simulink model "case3"  (R2024b)
settings: Solver=FixedStepAuto  StartTime=0  StopTime=1  FixedStep=1e-7  RelTol=1e-3
values from neighbouring files (symbols this model uses):
  SG_D_1_D = 0.01056    [IEEE9_case_parameters.m]    (also in case1_parameters.m; case2_parameters.m; case3_parameters.m; case4_parameters.m)
  SG_D_1_EnableSaturation = 0    [IEEE9_case_parameters.m]    (also in case1_parameters.m; case2_parameters.m; case3_parameters.m; case4_parameters.m)
  SG_D_1_f0 = 60    [IEEE9_case_parameters.m]    (also in case1_parameters.m; case2_parameters.m; case3_parameters.m; case4_parameters.m)
  SG_D_1_H = 7.5    [IEEE9_case_parameters.m]    (also in case1_parameters.m; case2_parameters.m; case3_parameters.m; case4_parameters.m)
  SG_D_1_K_A = 20    [IEEE9_case_parameters.m]    (also in case1_parameters.m; case2_parameters.m; case3_parameters.m; case4_parameters.m)
  SG_D_1_K_E = 1.000000e+1    (= 10)    [IEEE9_case_parameters.m]    (also in case1_parameters.m; case2_parameters.m; case3_parameters.m; case4_parameters.m)
  SG_D_1_K_F = 2.363    [IEEE9_case_parameters.m]    (also in case1_parameters.m; case2_parameters.m; case3_parameters.m; case4_parameters.m)
  SG_D_1_K_s = 0.5    [IEEE9_case_parameters.m]    (also in case1_parameters.m = 5; case2_parameters.m = 5; case3_parameters.m = 5; case4_parameters.m = 5)
  SG_D_1_R_a = 0.001088    [IEEE9_case_parameters.m]    (also in case1_parameters.m; case2_parameters.m; case3_parameters.m; case4_parameters.m)
  SG_D_1_S_A = 1    [IEEE9_case_parameters.m]    (also in case1_parameters.m; case2_parameters.m; case3_parameters.m; case4_parameters.m)
  SG_D_1_S_B = 0.103    [IEEE9_case_parameters.m]    (also in case1_parameters.m; case2_parameters.m; case3_parameters.m; case4_parameters.m)
  SG_D_1_S_N = 10.659857    [IEEE9_case_parameters.m]    (also in case1_parameters.m; case2_parameters.m; case3_parameters.m; case4_parameters.m)
  SG_D_1_SpeedPara = 200    [IEEE9_case_parameters.m]    (also in case1_parameters.m; case2_parameters.m; case3_parameters.m; case4_parameters.m)
  SG_D_1_T_0 = 0.720173    [IEEE9_case_parameters.m]    (also in case1_parameters.m = 0.755522; case2_parameters.m = 0.808931; case3_parameters.m = 0.869402; case4_parameters.m = 0.729316)
  SG_D_1_T_1 = 0.3    [IEEE9_case_parameters.m]    (also in case1_parameters.m; case2_parameters.m; case3_parameters.m; case4_parameters.m)
  SG_D_1_T_2 = 0.05    [IEEE9_case_parameters.m]    (also in case1_parameters.m; case2_parameters.m; case3_parameters.m; case4_parameters.m)
  SG_D_1_T_3 = 0.02    [IEEE9_case_parameters.m]    (also in case1_parameters.m; case2_parameters.m; case3_parameters.m; case4_parameters.m)
  SG_D_1_T_4 = 0.005    [IEEE9_case_parameters.m]    (also in case1_parameters.m; case2_parameters.m; case3_parameters.m; case4_parameters.m)
  SG_D_1_T_A = 0.02    [IEEE9_case_parameters.m]    (also in case1_parameters.m; case2_parameters.m; case3_parameters.m; case4_parameters.m)
  SG_D_1_T_dd = 8.000000e+0    (= 8)    [IEEE9_case_parameters.m]    (also in case1_parameters.m; case2_parameters.m; case3_parameters.m; case4_parameters.m)
  SG_D_1_T_ddd = 0.04    [IEEE9_case_parameters.m]    (also in case1_parameters.m; case2_parameters.m; case3_parameters.m; case4_parameters.m)
  SG_D_1_T_E = 0.314    [IEEE9_case_parameters.m]    (also in case1_parameters.m; case2_parameters.m; case3_parameters.m; case4_parameters.m)
  SG_D_1_T_F = 0.35    [IEEE9_case_parameters.m]    (also in case1_parameters.m; case2_parameters.m; case3_parameters.m; case4_parameters.m)
  SG_D_1_T_qd = 0.8    [IEEE9_case_parameters.m]    (also in case1_parameters.m; case2_parameters.m; case3_parameters.m; case4_parameters.m)
  SG_D_1_T_qdd = 0.02    [IEEE9_case_parameters.m]    (also in case1_parameters.m; case2_parameters.m; case3_parameters.m; case4_parameters.m)
  SG_D_1_T_speed = 0.1    [IEEE9_case_parameters.m]    (also in case1_parameters.m = 200; case2_parameters.m = 200; case3_parameters.m = 200; case4_parameters.m = 200)
  SG_D_1_T_w = 0.5    [IEEE9_case_parameters.m]    (also in case1_parameters.m; case2_parameters.m; case3_parameters.m; case4_parameters.m)
  SG_D_1_V_ref = 1.990276    [IEEE9_case_parameters.m]    (also in case1_parameters.m = 2.042296; case2_parameters.m = 2.051388; case3_parameters.m = 2.089584; case4_parameters.m = 2.01845)
  SG_D_1_w_ref = 376.991118    [IEEE9_case_parameters.m]    (also in case1_parameters.m; case2_parameters.m; case3_parameters.m; case4_parameters.m)
  SG_D_1_wb = 6.000000e+1    (= 60)    [IEEE9_case_parameters.m]    (also in case1_parameters.m; case2_parameters.m; case3_parameters.m; case4_parameters.m)
  SG_D_1_x_d = 1.9    [IEEE9_case_parameters.m]    (also in case1_parameters.m; case2_parameters.m; case3_parameters.m; case4_parameters.m)
  SG_D_1_x_dd = 0.302    [IEEE9_case_parameters.m]    (also in case1_parameters.m; case2_parameters.m; case3_parameters.m; case4_parameters.m)
  SG_D_1_x_ddd = 0.204    [IEEE9_case_parameters.m]    (also in case1_parameters.m; case2_parameters.m; case3_parameters.m; case4_parameters.m)
  SG_D_1_x_l = 0.05    [IEEE9_case_parameters.m]    (also in case1_parameters.m; case2_parameters.m; case3_parameters.m; case4_parameters.m)
  SG_D_1_x_q = 1.3    [IEEE9_case_parameters.m]    (also in case1_parameters.m; case2_parameters.m; case3_parameters.m; case4_parameters.m)
  SG_D_1_x_qd = 0.5    [IEEE9_case_parameters.m]    (also in case1_parameters.m; case2_parameters.m; case3_parameters.m; case4_parameters.m)
  SG_D_1_x_qdd = 0.3    [IEEE9_case_parameters.m]    (also in case1_parameters.m; case2_parameters.m; case3_parameters.m; case4_parameters.m)
  SG_D_2_D = 0.02    [IEEE9_case_parameters.m]    (also in case1_parameters.m; case2_parameters.m; case3_parameters.m; case4_parameters.m)
  SG_D_2_EnableSaturation = 0    [IEEE9_case_parameters.m]    (also in case1_parameters.m; case2_parameters.m; case3_parameters.m; case4_parameters.m)
  SG_D_2_f0 = 60    [IEEE9_case_parameters.m]    (also in case1_parameters.m; case2_parameters.m; case3_parameters.m; case4_parameters.m)
  SG_D_2_H = 8.000000e+0    (= 8)    [IEEE9_case_parameters.m]    (also in case1_parameters.m; case2_parameters.m; case3_parameters.m; case4_parameters.m)
  SG_D_2_K_A = 20    [IEEE9_case_parameters.m]    (also in case1_parameters.m; case2_parameters.m; case3_parameters.m; case4_parameters.m)
  SG_D_2_K_E = 1.000000e+1    (= 10)    [IEEE9_case_parameters.m]    (also in case1_parameters.m; case2_parameters.m; case3_parameters.m; case4_parameters.m)
  SG_D_2_K_F = 2.363    [IEEE9_case_parameters.m]    (also in case1_parameters.m; case2_parameters.m; case3_parameters.m; case4_parameters.m)
  SG_D_2_K_s = 0.5    [IEEE9_case_parameters.m]    (also in case1_parameters.m = 4; case2_parameters.m = 4; case3_parameters.m = 4; case4_parameters.m = 4)
  SG_D_2_R_a = 0.001088    [IEEE9_case_parameters.m]    (also in case1_parameters.m; case2_parameters.m; case3_parameters.m; case4_parameters.m)
  SG_D_2_S_A = 1    [IEEE9_case_parameters.m]    (also in case1_parameters.m; case2_parameters.m; case3_parameters.m; case4_parameters.m)
  SG_D_2_S_B = 0.103    [IEEE9_case_parameters.m]    (also in case1_parameters.m; case2_parameters.m; case3_parameters.m; case4_parameters.m)
  SG_D_2_S_N = 10.659857    [IEEE9_case_parameters.m]    (also in case1_parameters.m; case2_parameters.m; case3_parameters.m; case4_parameters.m)
  SG_D_2_SpeedPara = 200    [IEEE9_case_parameters.m]    (also in case1_parameters.m; case2_parameters.m; case3_parameters.m; case4_parameters.m)
  SG_D_2_T_0 = 1.632913    [IEEE9_case_parameters.m]    (also in case1_parameters.m = 1.632925; case2_parameters.m = 1.632915; case3_parameters.m = 1.632914; case4_parameters.m = 1.632927)
  SG_D_2_T_1 = 0.2    [IEEE9_case_parameters.m]    (also in case1_parameters.m; case2_parameters.m; case3_parameters.m; case4_parameters.m)
  SG_D_2_T_2 = 0.05    [IEEE9_case_parameters.m]    (also in case1_parameters.m; case2_parameters.m; case3_parameters.m; case4_parameters.m)
  SG_D_2_T_3 = 0.02    [IEEE9_case_parameters.m]    (also in case1_parameters.m; case2_parameters.m; case3_parameters.m; case4_parameters.m)
  SG_D_2_T_4 = 0.005    [IEEE9_case_parameters.m]    (also in case1_parameters.m; case2_parameters.m; case3_parameters.m; case4_parameters.m)
  SG_D_2_T_A = 0.02    [IEEE9_case_parameters.m]    (also in case1_parameters.m; case2_parameters.m; case3_parameters.m; case4_parameters.m)
  SG_D_2_T_dd = 7.9    [IEEE9_case_parameters.m]    (also in case1_parameters.m; case2_parameters.m; case3_parameters.m; case4_parameters.m)
  SG_D_2_T_ddd = 0.04    [IEEE9_case_parameters.m]    (also in case1_parameters.m; case2_parameters.m; case3_parameters.m; case4_parameters.m)
  SG_D_2_T_E = 0.314    [IEEE9_case_parameters.m]    (also in case1_parameters.m; case2_parameters.m; case3_parameters.m; case4_parameters.m)
  SG_D_2_T_F = 0.35    [IEEE9_case_parameters.m]    (also in case1_parameters.m; case2_parameters.m; case3_parameters.m; case4_parameters.m)
  SG_D_2_T_qd = 0.8    [IEEE9_case_parameters.m]    (also in case1_parameters.m; case2_parameters.m; case3_parameters.m; case4_parameters.m)
  SG_D_2_T_qdd = 0.015    [IEEE9_case_parameters.m]    (also in case1_parameters.m; case2_parameters.m; case3_parameters.m; case4_parameters.m)
  SG_D_2_T_speed = 0.1    [IEEE9_case_parameters.m]    (also in case1_parameters.m = 150; case2_parameters.m = 150; case3_parameters.m = 150; case4_parameters.m = 150)
  SG_D_2_T_w = 0.35    [IEEE9_case_parameters.m]    (also in case1_parameters.m; case2_parameters.m; case3_parameters.m; case4_parameters.m)
  SG_D_2_V_ref = 2.58547    [IEEE9_case_parameters.m]    (also in case1_parameters.m = 2.597896; case2_parameters.m = 2.587136; case3_parameters.m = 2.586042; case4_parameters.m = 2.599679)
  SG_D_2_w_ref = 376.991118    [IEEE9_case_parameters.m]    (also in case1_parameters.m; case2_parameters.m; case3_parameters.m; case4_parameters.m)
  SG_D_2_wb = 6.000000e+1    (= 60)    [IEEE9_case_parameters.m]    (also in case1_parameters.m; case2_parameters.m; case3_parameters.m; case4_parameters.m)
  SG_D_2_x_d = 1.8    [IEEE9_case_parameters.m]    (also in case1_parameters.m; case2_parameters.m; case3_parameters.m; case4_parameters.m)
  SG_D_2_x_dd = 0.302    [IEEE9_case_parameters.m]    (also in case1_parameters.m; case2_parameters.m; case3_parameters.m; case4_parameters.m)
  SG_D_2_x_ddd = 0.204    [IEEE9_case_parameters.m]    (also in case1_parameters.m; case2_parameters.m; case3_parameters.m; case4_parameters.m)
  SG_D_2_x_l = 0.05    [IEEE9_case_parameters.m]    (also in case1_parameters.m; case2_parameters.m; case3_parameters.m; case4_parameters.m)
  SG_D_2_x_q = 1.25    [IEEE9_case_parameters.m]    (also in case1_parameters.m; case2_parameters.m; case3_parameters.m; case4_parameters.m)
  SG_D_2_x_qd = 0.5    [IEEE9_case_parameters.m]    (also in case1_parameters.m; case2_parameters.m; case3_parameters.m; case4_parameters.m)
  SG_D_2_x_qdd = 0.3    [IEEE9_case_parameters.m]    (also in case1_parameters.m; case2_parameters.m; case3_parameters.m; case4_parameters.m)
  SG_D_3_D = 0.02    [IEEE9_case_parameters.m]    (also in case1_parameters.m; case2_parameters.m; case3_parameters.m; case4_parameters.m)
  SG_D_3_EnableSaturation = 0    [IEEE9_case_parameters.m]    (also in case1_parameters.m; case2_parameters.m; case3_parameters.m; case4_parameters.m)
  SG_D_3_f0 = 60    [IEEE9_case_parameters.m]    (also in case1_parameters.m; case2_parameters.m; case3_parameters.m; case4_parameters.m)
  SG_D_3_H = 7.7    [IEEE9_case_parameters.m]    (also in case1_parameters.m; case2_parameters.m; case3_parameters.m; case4_parameters.m)
  SG_D_3_K_A = 20    [IEEE9_case_parameters.m]    (also in case1_parameters.m; case2_parameters.m; case3_parameters.m; case4_parameters.m)
  SG_D_3_K_E = 1.000000e+1    (= 10)    [IEEE9_case_parameters.m]    (also in case1_parameters.m; case2_parameters.m; case3_parameters.m; case4_parameters.m)
  SG_D_3_K_F = 2.363    [IEEE9_case_parameters.m]    (also in case1_parameters.m; case2_parameters.m; case3_parameters.m; case4_parameters.m)
  SG_D_3_K_s = 0.2    [IEEE9_case_parameters.m]    (also in case1_parameters.m = 2; case2_parameters.m = 2; case3_parameters.m = 2; case4_parameters.m = 2)
  SG_D_3_R_a = 0.001088    [IEEE9_case_parameters.m]    (also in case1_parameters.m; case2_parameters.m; case3_parameters.m; case4_parameters.m)
  SG_D_3_S_A = 1    [IEEE9_case_parameters.m]    (also in case1_parameters.m; case2_parameters.m; case3_parameters.m; case4_parameters.m)
  SG_D_3_S_B = 0.103    [IEEE9_case_parameters.m]    (also in case1_parameters.m; case2_parameters.m; case3_parameters.m; case4_parameters.m)
  SG_D_3_S_N = 10.659857    [IEEE9_case_parameters.m]    (also in case1_parameters.m; case2_parameters.m; case3_parameters.m; case4_parameters.m)
  SG_D_3_SpeedPara = 200    [IEEE9_case_parameters.m]    (also in case1_parameters.m; case2_parameters.m; case3_parameters.m; case4_parameters.m)
  SG_D_3_T_0 = 0.850788    [IEEE9_case_parameters.m]    (also in case1_parameters.m = 0.850786; case2_parameters.m = 0.850787; case3_parameters.m; case4_parameters.m = 0.850786)
  SG_D_3_T_1 = 0.2    [IEEE9_case_parameters.m]    (also in case1_parameters.m; case2_parameters.m; case3_parameters.m; case4_parameters.m)
  SG_D_3_T_2 = 0.05    [IEEE9_case_parameters.m]    (also in case1_parameters.m; case2_parameters.m; case3_parameters.m; case4_parameters.m)
  SG_D_3_T_3 = 0.02    [IEEE9_case_parameters.m]    (also in case1_parameters.m; case2_parameters.m; case3_parameters.m; case4_parameters.m)
  SG_D_3_T_4 = 0.005    [IEEE9_case_parameters.m]    (also in case1_parameters.m; case2_parameters.m; case3_parameters.m; case4_parameters.m)
  SG_D_3_T_A = 0.02    [IEEE9_case_parameters.m]    (also in case1_parameters.m; case2_parameters.m; case3_parameters.m; case4_parameters.m)
  SG_D_3_T_dd = 8.1    [IEEE9_case_parameters.m]    (also in case1_parameters.m; case2_parameters.m; case3_parameters.m; case4_parameters.m)
  SG_D_3_T_ddd = 0.04    [IEEE9_case_parameters.m]    (also in case1_parameters.m; case2_parameters.m; case3_parameters.m; case4_parameters.m)
  SG_D_3_T_E = 0.314    [IEEE9_case_parameters.m]    (also in case1_parameters.m; case2_parameters.m; case3_parameters.m; case4_parameters.m)
  SG_D_3_T_F = 0.35    [IEEE9_case_parameters.m]    (also in case1_parameters.m; case2_parameters.m; case3_parameters.m; case4_parameters.m)
  SG_D_3_T_qd = 0.8    [IEEE9_case_parameters.m]    (also in case1_parameters.m; case2_parameters.m; case3_parameters.m; case4_parameters.m)
  SG_D_3_T_qdd = 0.015    [IEEE9_case_parameters.m]    (also in case1_parameters.m; case2_parameters.m; case3_parameters.m; case4_parameters.m)
  SG_D_3_T_speed = 0.1    [IEEE9_case_parameters.m]    (also in case1_parameters.m = 180; case2_parameters.m = 180; case3_parameters.m = 180; case4_parameters.m = 180)
  SG_D_3_T_w = 0.4    [IEEE9_case_parameters.m]    (also in case1_parameters.m; case2_parameters.m; case3_parameters.m; case4_parameters.m)
  SG_D_3_V_ref = 1.892727    [IEEE9_case_parameters.m]    (also in case1_parameters.m = 1.906439; case2_parameters.m = 1.895535; case3_parameters.m = 1.892105; case4_parameters.m = 1.906598)
  SG_D_3_w_ref = 376.991118    [IEEE9_case_parameters.m]    (also in case1_parameters.m; case2_parameters.m; case3_parameters.m; case4_parameters.m)
  SG_D_3_wb = 6.000000e+1    (= 60)    [IEEE9_case_parameters.m]    (also in case1_parameters.m; case2_parameters.m; case3_parameters.m; case4_parameters.m)
  SG_D_3_x_d = 1.85    [IEEE9_case_parameters.m]    (also in case1_parameters.m; case2_parameters.m; case3_parameters.m; case4_parameters.m)
  SG_D_3_x_dd = 0.302    [IEEE9_case_parameters.m]    (also in case1_parameters.m; case2_parameters.m; case3_parameters.m; case4_parameters.m)
  SG_D_3_x_ddd = 0.204    [IEEE9_case_parameters.m]    (also in case1_parameters.m; case2_parameters.m; case3_parameters.m; case4_parameters.m)
  SG_D_3_x_l = 0.05    [IEEE9_case_parameters.m]    (also in case1_parameters.m; case2_parameters.m; case3_parameters.m; case4_parameters.m)
  SG_D_3_x_q = 1.2    [IEEE9_case_parameters.m]    (also in case1_parameters.m; case2_parameters.m; case3_parameters.m; case4_parameters.m)
  SG_D_3_x_qd = 0.5    [IEEE9_case_parameters.m]    (also in case1_parameters.m; case2_parameters.m; case3_parameters.m; case4_parameters.m)
  SG_D_3_x_qdd = 0.3    [IEEE9_case_parameters.m]    (also in case1_parameters.m; case2_parameters.m; case3_parameters.m; case4_parameters.m)
(part 7 of 12)

== system case3/SG_D_2/T_e_SG_D_2_block ==
  note: T_e_SG_D_2 in case3
      | $-\frac{\psi _{d,\mathrm{SG},D,2}\,\left(\psi _{q,\mathrm{SG},D,2}+\frac{\psi _{\mathrm{gq},\mathrm{SG},D,2}\,\left(x_{l}-x_{\mathrm{qdd}}\right)}{x_{l}-x_{\mathrm{qd}}}+\frac{\psi _{\mathrm{kq},\mathrm{SG},D,2}\,\left(x_{\mathrm{qd}}-x_{\mathrm{qdd}}\right)}{x_{l}-x_{\mathrm{qd}}}\right)}{x_{\mathrm{qdd}}}-\frac{\psi _{q,\mathrm{SG},D,2}\,\left(\frac{\psi _{\mathrm{1d},\mathrm{SG},D,2}\,\left(x_{\mathrm{dd}}-x_{\mathrm{ddd}}\right)}{x_{\mathrm{dd}}-x_{l}}-\psi _{d,\mathrm{SG},D,2}+\frac{\psi _{\mathrm{fd},\mathrm{SG},D,2}\,\left(x_{\mathrm{ddd}}-x_{l}\right)}{x_{\mathrm{dd}}-x_{l}}\right)}{x_{\mathrm{ddd}}}$
      | Automatically generated on 2025-10-31 19:00:41 .
  State_psi_d_SG_D_2_bd8f2 : Inport
  State_psi_gq_SG_D_2_7cf1b : Inport  Port=2
  State_psi_kq_SG_D_2_00a62 : Inport  Port=3
  State_psi_q_SG_D_2_fc5b5 : Inport  Port=4
  State_psi_q_SG_D_2_0409e : Inport  Port=5
  State_psi_1d_SG_D_2_3067b : Inport  Port=6
  State_psi_d_SG_D_2_0f14f : Inport  Port=7
  State_psi_fd_SG_D_2_e1184 : Inport  Port=8
  Add_1d177 : Sum
  Add_42747 : Sum
  Add_5d270 : Sum
  Add_b1493 : Sum
  Add_c9106 : Sum
  Add_e7ab1 : Sum
  Constant_-1_0d88f : Constant  Value=-1
  Constant_-1_2e7fe : Constant  Value=-1
  Constant_-1_4cbe8 : Constant  Value=-1
  Constant_-1_6ebdc : Constant  Value=-1
  Constant_-1_f2e90 : Constant  Value=-1
  Constant_x_dd_7ba48 : Constant  Value=x_dd
  Constant_x_dd_9e0e7 : Constant  Value=x_dd
  Constant_x_dd_a49ec : Constant  Value=x_dd
  Constant_x_ddd_3889b : Constant  Value=x_ddd
  Constant_x_ddd_8a46c : Constant  Value=x_ddd
  Constant_x_ddd_f7651 : Constant  Value=x_ddd
  Constant_x_l_2e2bb : Constant  Value=x_l
  Constant_x_l_3f6eb : Constant  Value=x_l
  Constant_x_l_47e81 : Constant  Value=x_l
  Constant_x_l_4ea90 : Constant  Value=x_l
  Constant_x_l_7f158 : Constant  Value=x_l
  Constant_x_l_d88ad : Constant  Value=x_l
  Constant_x_qd_2c9ed : Constant  Value=x_qd
  Constant_x_qd_5af5b : Constant  Value=x_qd
  Constant_x_qd_fa8b9 : Constant  Value=x_qd
  Constant_x_qdd_6bb06 : Constant  Value=x_qdd
  Constant_x_qdd_71248 : Constant  Value=x_qdd
  Constant_x_qdd_ce159 : Constant  Value=x_qdd
  Divide_3e111 : Product  Inputs=*/
  Divide_4e959 : Product  Inputs=*/
  Divide_66ff5 : Product  Inputs=*/
  Divide_7bee8 : Product  Inputs=*/
  Divide_7d3ab : Product  Inputs=*/
  Divide_8540e : Product  Inputs=*/
  Product_2024f : Product
  Product_2debf : Product
  Product_312dd : Product
  Product_42b1c : Product
  Product_56005 : Product
  Product_711bf : Product
  Product_73a18 : Product
  Product_b399e : Product
  Product_bcb12 : Product
  Product_e72c3 : Product
  Product_f0df5 : Product
  Subtract_1307a : Sum  Inputs=+-
  Subtract_1559b : Sum  Inputs=+-
  Subtract_45dc1 : Sum  Inputs=+-
  Subtract_73649 : Sum  Inputs=+-
  Subtract_9e724 : Sum  Inputs=+-
  Subtract_cfab8 : Sum  Inputs=+-
  Subtract_da0d6 : Sum  Inputs=+-
  Blockout_T_e_SG_D_2_f9887 : Outport
  wires:
  Constant_-1_6ebdc/1 -> Product_bcb12/1
  Divide_7d3ab/1 -> Subtract_cfab8/1
  Constant_-1_4cbe8/1 -> Product_73a18/1
  Constant_x_l_3f6eb/1 -> Product_73a18/2
  Constant_x_qd_5af5b/1 -> Subtract_da0d6/1
  Product_e72c3/1 -> Divide_7d3ab/1
  Product_73a18/1 -> Add_e7ab1/1
  Divide_7bee8/1 -> Subtract_9e724/2
  Constant_x_qdd_71248/1 -> Subtract_da0d6/2
  Constant_x_qdd_6bb06/1 -> Divide_66ff5/2
  Constant_x_ddd_8a46c/1 -> Subtract_73649/2
  Constant_x_qdd_ce159/1 -> Add_e7ab1/2
  Constant_x_l_47e81/1 -> Product_bcb12/2
  Constant_-1_f2e90/1 -> Product_2debf/1
  Constant_x_l_7f158/1 -> Product_2debf/2
  Constant_-1_0d88f/1 -> Product_b399e/1
  State_psi_1d_SG_D_2_3067b/1 -> Product_b399e/2
  Constant_x_dd_9e0e7/1 -> Subtract_73649/1
  Divide_8540e/1 -> Subtract_cfab8/2
  State_psi_gq_SG_D_2_7cf1b/1 -> Product_e72c3/1
  Add_e7ab1/1 -> Product_e72c3/2
  Subtract_cfab8/1 -> Add_5d270/1
  Constant_x_dd_7ba48/1 -> Subtract_45dc1/1
  Product_bcb12/1 -> Add_c9106/1
  Product_56005/1 -> Product_2024f/1
  Constant_x_qd_fa8b9/1 -> Add_c9106/2
  State_psi_kq_SG_D_2_00a62/1 -> Product_312dd/1
  Subtract_da0d6/1 -> Product_312dd/2
  Product_2debf/1 -> Add_b1493/1
  State_psi_q_SG_D_2_0409e/1 -> Product_42b1c/1
  Constant_x_qd_2c9ed/1 -> Add_b1493/2
  Product_b399e/1 -> Product_711bf/1
  Divide_4e959/1 -> Add_42747/2
  Subtract_73649/1 -> Product_711bf/2
  Constant_x_l_d88ad/1 -> Subtract_45dc1/2
  Constant_x_ddd_3889b/1 -> Subtract_1307a/1
  Constant_x_dd_a49ec/1 -> Subtract_1559b/1
  Constant_x_l_2e2bb/1 -> Subtract_1307a/2
  Add_42747/1 -> Blockout_T_e_SG_D_2_f9887/1
  Add_c9106/1 -> Divide_7d3ab/2
  Product_312dd/1 -> Divide_8540e/1
  Product_2024f/1 -> Divide_66ff5/1
  State_psi_d_SG_D_2_bd8f2/1 -> Product_56005/2
  Add_b1493/1 -> Divide_8540e/2
  Product_711bf/1 -> Divide_3e111/1
  Subtract_45dc1/1 -> Divide_3e111/2
  Constant_x_l_4ea90/1 -> Subtract_1559b/2
  State_psi_fd_SG_D_2_e1184/1 -> Product_f0df5/1
  Constant_x_ddd_f7651/1 -> Divide_4e959/2
  Product_42b1c/1 -> Divide_4e959/1
  Subtract_1307a/1 -> Product_f0df5/2
  Divide_3e111/1 -> Add_1d177/1
  State_psi_d_SG_D_2_0f14f/1 -> Add_1d177/2
  Add_1d177/1 -> Subtract_9e724/1
  Product_f0df5/1 -> Divide_7bee8/1
  Subtract_1559b/1 -> Divide_7bee8/2
  Constant_-1_2e7fe/1 -> Product_56005/1
  State_psi_q_SG_D_2_fc5b5/1 -> Add_5d270/2
  Add_5d270/1 -> Product_2024f/2
  Subtract_9e724/1 -> Product_42b1c/2
  Divide_66ff5/1 -> Add_42747/1

== system case3/SG_D_2/d_E_fd_SG_D_2_block ==
  note: d_E_fd_SG_D_2 in case3
      | $\frac{V_{f,\mathrm{SG},D,2}-E_{\mathrm{fd},\mathrm{SG},D,2}\,K_{E}}{T_{E}}$
      | Automatically generated on 2025-10-31 19:00:25 .
  State_E_fd_SG_D_2_aeb78 : Inport
  State_V_f_SG_D_2_75a88 : Inport  Port=2
  Add_3aad2 : Sum
  Constant_-1_2bcf9 : Constant  Value=-1
  Constant_K_E_34ed1 : Constant  Value=K_E
  Constant_T_E_1a99d : Constant  Value=T_E
  Divide_16824 : Product  Inputs=*/
  Product_22060 : Product
  Product_ea532 : Product
  Blockout_d_E_fd_SG_D_2_c4f8a : Outport
  wires:
  Constant_-1_2bcf9/1 -> Product_ea532/1
  State_E_fd_SG_D_2_aeb78/1 -> Product_ea532/2
  Product_ea532/1 -> Product_22060/1
  Constant_K_E_34ed1/1 -> Product_22060/2
  Product_22060/1 -> Add_3aad2/1
  Constant_T_E_1a99d/1 -> Divide_16824/2
  State_V_f_SG_D_2_75a88/1 -> Add_3aad2/2
  Add_3aad2/1 -> Divide_16824/1
  Divide_16824/1 -> Blockout_d_E_fd_SG_D_2_c4f8a/1

== system case3/SG_D_2/d_Px_1_SG_D_2_block ==
  note: d_Px_1_SG_D_2 in case3
      | $\frac{w_{\mathrm{SG},D,2}-2\,\pi \,f_{0}}{T_{w}}-\frac{\mathrm{Px}_{1,\mathrm{SG},D,2}}{T_{w}}$
      | Automatically generated on 2025-10-31 19:00:26 .
  State_Px_1_SG_D_2_e1673 : Inport
  State_w_SG_D_2_bbb39 : Inport  Port=2
  Add_08d45 : Sum
  Add_4d18d : Sum
  Constant_-1_0bff0 : Constant  Value=-1
  Constant_-2.0_0421e : Constant  Value=-2.0
  Constant_T_w_34646 : Constant  Value=T_w
  Constant_T_w_c89ad : Constant  Value=T_w
  Constant_f0_04b6a : Constant  Value=f0
  Constant_pi_beef7 : Constant  Value=pi
  Divide_48226 : Product  Inputs=*/
  Divide_d9862 : Product  Inputs=*/
  Product_7dcbd : Product
  Product_cef66 : Product
  Product_ec7ca : Product
  Blockout_d_Px_1_SG_D_2_109b7 : Outport
  wires:
  Constant_-2.0_0421e/1 -> Product_7dcbd/1
  State_w_SG_D_2_bbb39/1 -> Add_4d18d/2
  Constant_pi_beef7/1 -> Product_7dcbd/2
  Product_7dcbd/1 -> Product_ec7ca/1
  Constant_f0_04b6a/1 -> Product_ec7ca/2
  Constant_-1_0bff0/1 -> Product_cef66/1
  State_Px_1_SG_D_2_e1673/1 -> Product_cef66/2
  Product_ec7ca/1 -> Add_4d18d/1
  Product_cef66/1 -> Divide_48226/1
  Constant_T_w_c89ad/1 -> Divide_48226/2
  Add_4d18d/1 -> Divide_d9862/1
  Constant_T_w_34646/1 -> Divide_d9862/2
  Divide_48226/1 -> Add_08d45/1
  Divide_d9862/1 -> Add_08d45/2
  Add_08d45/1 -> Blockout_d_Px_1_SG_D_2_109b7/1

== system case3/SG_D_2/d_Px_2_SG_D_2_block ==
  note: d_Px_2_SG_D_2 in case3
      | $\frac{\mathrm{Px}_{1,\mathrm{SG},D,2}-T_{2}\,\left(\frac{\mathrm{Px}_{1,\mathrm{SG},D,2}}{T_{w}}-\frac{w_{\mathrm{SG},D,2}-2\,\pi \,f_{0}}{T_{w}}\right)}{T_{1}}-\frac{\mathrm{Px}_{2,\mathrm{SG},D,2}}{T_{1}}$
      | Automatically generated on 2025-10-31 19:00:27 .
  State_Px_2_SG_D_2_a9fab : Inport
  State_Px_1_SG_D_2_b7eac : Inport  Port=2
  State_Px_1_SG_D_2_ca2a4 : Inport  Port=3
  State_w_SG_D_2_0d46f : Inport  Port=4
  Add_05522 : Sum
  Add_5cdaa : Sum
  Add_6c463 : Sum
  Add_d61f3 : Sum
  Constant_-1_14cce : Constant  Value=-1
  Constant_-1_44d6b : Constant  Value=-1
  Constant_-2.0_02914 : Constant  Value=-2.0
  Constant_T_1_53e96 : Constant  Value=T_1
  Constant_T_1_a5862 : Constant  Value=T_1
  Constant_T_2_b2b5a : Constant  Value=T_2
  Constant_T_w_a3a65 : Constant  Value=T_w
  Constant_T_w_e47eb : Constant  Value=T_w
  Constant_f0_8ff7e : Constant  Value=f0
  Constant_pi_131b0 : Constant  Value=pi
  Divide_9619a : Product  Inputs=*/
  Divide_a2959 : Product  Inputs=*/
  Divide_bb976 : Product  Inputs=*/
  Divide_df334 : Product  Inputs=*/
  Product_334ce : Product
  Product_6f84f : Product
  Product_de7e1 : Product
  Product_ed4b0 : Product
  Product_f3691 : Product
  Blockout_d_Px_2_SG_D_2_1ade1 : Outport
  wires:
  Constant_-1_14cce/1 -> Product_334ce/1
  Constant_-2.0_02914/1 -> Product_de7e1/1
  Product_f3691/1 -> Add_5cdaa/2
  State_w_SG_D_2_0d46f/1 -> Add_6c463/2
  Constant_pi_131b0/1 -> Product_de7e1/2
  Product_de7e1/1 -> Product_ed4b0/1
  State_Px_1_SG_D_2_ca2a4/1 -> Product_6f84f/2
  Constant_f0_8ff7e/1 -> Product_ed4b0/2
  State_Px_2_SG_D_2_a9fab/1 -> Product_334ce/2
  Constant_-1_44d6b/1 -> Product_6f84f/1
  Product_ed4b0/1 -> Add_6c463/1
  Product_6f84f/1 -> Divide_a2959/1
  Constant_T_w_a3a65/1 -> Divide_a2959/2
  Add_6c463/1 -> Divide_9619a/1
  Constant_T_w_e47eb/1 -> Divide_9619a/2
  Divide_a2959/1 -> Add_05522/1
  Divide_9619a/1 -> Add_05522/2
  Constant_T_2_b2b5a/1 -> Product_f3691/1
  Add_05522/1 -> Product_f3691/2
  State_Px_1_SG_D_2_b7eac/1 -> Add_5cdaa/1
  Product_334ce/1 -> Divide_df334/1
  Constant_T_1_a5862/1 -> Divide_df334/2
  Add_5cdaa/1 -> Divide_bb976/1
  Constant_T_1_53e96/1 -> Divide_bb976/2
  Divide_df334/1 -> Add_d61f3/1
  Divide_bb976/1 -> Add_d61f3/2
  Add_d61f3/1 -> Blockout_d_Px_2_SG_D_2_1ade1/1

== system case3/SG_D_2/d_Px_3_SG_D_2_block ==
  note: d_Px_3_SG_D_2 in case3
      | $\frac{\mathrm{Px}_{2,\mathrm{SG},D,2}+T_{4}\,\left(\frac{\mathrm{Px}_{1,\mathrm{SG},D,2}-T_{2}\,\left(\frac{\mathrm{Px}_{1,\mathrm{SG},D,2}}{T_{w}}-\frac{w_{\mathrm{SG},D,2}-2\,\pi \,f_{0}}{T_{w}}\right)}{T_{1}}-\frac{\mathrm{Px}_{2,\mathrm{SG},D,2}}{T_{1}}\right)}{T_{3}}-\frac{\mathrm{Px}_{3,\mathrm{SG},D,2}}{T_{3}}$
      | Automatically generated on 2025-10-31 19:00:30 .
  State_Px_3_SG_D_2_127e3 : Inport
  State_Px_2_SG_D_2_c1187 : Inport  Port=2
  State_Px_2_SG_D_2_e6f9b : Inport  Port=3
  State_Px_1_SG_D_2_d9778 : Inport  Port=4
  State_Px_1_SG_D_2_e27f8 : Inport  Port=5
  State_w_SG_D_2_22dc6 : Inport  Port=6
  Add_0cd75 : Sum
  Add_9f753 : Sum
  Add_ad80e : Sum
  Add_bc041 : Sum
  Add_d454c : Sum
  Add_e63a9 : Sum
  Constant_-1_07edb : Constant  Value=-1
  Constant_-1_13db9 : Constant  Value=-1
  Constant_-1_77d78 : Constant  Value=-1
  Constant_-2.0_d8f8b : Constant  Value=-2.0
  Constant_T_1_8ecf8 : Constant  Value=T_1
  Constant_T_1_fad53 : Constant  Value=T_1
  Constant_T_2_f64fd : Constant  Value=T_2
  Constant_T_3_52c41 : Constant  Value=T_3
  Constant_T_3_a0ec5 : Constant  Value=T_3
  Constant_T_4_606e5 : Constant  Value=T_4
  Constant_T_w_319fe : Constant  Value=T_w
  Constant_T_w_36f52 : Constant  Value=T_w
  Constant_f0_07c30 : Constant  Value=f0
  Constant_pi_a9680 : Constant  Value=pi
  Divide_5bcdb : Product  Inputs=*/
  Divide_6b17f : Product  Inputs=*/
  Divide_ba923 : Product  Inputs=*/
  Divide_beeaf : Product  Inputs=*/
  Divide_c57bf : Product  Inputs=*/
  Divide_f497b : Product  Inputs=*/
  Product_147fa : Product
  Product_201e1 : Product
  Product_24bd8 : Product
  Product_26550 : Product
  Product_2e2b4 : Product
  Product_4511e : Product
  Product_f1616 : Product
  Blockout_d_Px_3_SG_D_2_2b25a : Outport
  wires:
  Constant_-2.0_d8f8b/1 -> Product_4511e/1
  State_w_SG_D_2_22dc6/1 -> Add_ad80e/2
  Add_d454c/1 -> Divide_6b17f/1
  Constant_pi_a9680/1 -> Product_4511e/2
  Constant_-1_07edb/1 -> Product_201e1/1
  Product_4511e/1 -> Product_f1616/1
  State_Px_2_SG_D_2_e6f9b/1 -> Product_201e1/2
  State_Px_1_SG_D_2_e27f8/1 -> Product_147fa/2
  Divide_6b17f/1 -> Add_0cd75/2
  Constant_f0_07c30/1 -> Product_f1616/2
  Constant_-1_13db9/1 -> Product_147fa/1
  Product_f1616/1 -> Add_ad80e/1
  Product_147fa/1 -> Divide_c57bf/1
  Constant_T_w_36f52/1 -> Divide_c57bf/2
  Divide_ba923/1 -> Add_0cd75/1
  Add_ad80e/1 -> Divide_f497b/1
  Product_24bd8/1 -> Add_bc041/2
  Constant_T_w_319fe/1 -> Divide_f497b/2
  Divide_c57bf/1 -> Add_9f753/1
  State_Px_1_SG_D_2_d9778/1 -> Add_bc041/1
  Divide_f497b/1 -> Add_9f753/2
  Constant_-1_77d78/1 -> Product_26550/1
  Constant_T_2_f64fd/1 -> Product_24bd8/1
  Add_9f753/1 -> Product_24bd8/2
  Product_201e1/1 -> Divide_5bcdb/1
  Constant_T_1_fad53/1 -> Divide_5bcdb/2
  Add_bc041/1 -> Divide_beeaf/1
  Constant_T_1_8ecf8/1 -> Divide_beeaf/2
  Divide_5bcdb/1 -> Add_e63a9/1
  Divide_beeaf/1 -> Add_e63a9/2
  Constant_T_4_606e5/1 -> Product_2e2b4/1
  Add_e63a9/1 -> Product_2e2b4/2
  State_Px_3_SG_D_2_127e3/1 -> Product_26550/2
  State_Px_2_SG_D_2_c1187/1 -> Add_d454c/1
  Product_2e2b4/1 -> Add_d454c/2
  Product_26550/1 -> Divide_ba923/1
  Constant_T_3_a0ec5/1 -> Divide_ba923/2
  Constant_T_3_52c41/1 -> Divide_6b17f/2
  Add_0cd75/1 -> Blockout_d_Px_3_SG_D_2_2b25a/1

== system case3/SG_D_2/d_R_f_SG_D_2_block ==
  note: d_R_f_SG_D_2 in case3
      | $-\frac{R_{f,\mathrm{SG},D,2}-\frac{E_{\mathrm{fd},\mathrm{SG},D,2}\,K_{F}}{T_{F}}}{T_{F}}$
      | Automatically generated on 2025-10-31 19:00:25 .
  State_E_fd_SG_D_2_79ff1 : Inport
  State_R_f_SG_D_2_45923 : Inport  Port=2
  Constant_K_F_d98cf : Constant  Value=K_F
  Constant_T_F_376ec : Constant  Value=T_F
  Constant_T_F_d88ed : Constant  Value=T_F
  Divide_355e7 : Product  Inputs=*/
  Divide_91a29 : Product  Inputs=*/
  Product_1d90d : Product
  Subtract_81797 : Sum  Inputs=+-
  Blockout_d_R_f_SG_D_2_d9bc5 : Outport
  wires:
  Constant_T_F_376ec/1 -> Divide_355e7/2
  State_E_fd_SG_D_2_79ff1/1 -> Product_1d90d/1
  Constant_K_F_d98cf/1 -> Product_1d90d/2
  State_R_f_SG_D_2_45923/1 -> Subtract_81797/2
  Product_1d90d/1 -> Divide_355e7/1
  Divide_355e7/1 -> Subtract_81797/1
  Constant_T_F_d88ed/1 -> Divide_91a29/2
  Subtract_81797/1 -> Divide_91a29/1
  Divide_91a29/1 -> Blockout_d_R_f_SG_D_2_d9bc5/1

== system case3/SG_D_2/d_T_m_SG_D_2_block ==
  note: d_T_m_SG_D_2 in case3
      | $-\frac{T_{m,\mathrm{SG},D,2}-T_{0}+\frac{\mathrm{SpeedPara}\,\left(w_{\mathrm{SG},D,2}-w_{\mathrm{ref}}\right)}{2\,f_{0}\,\pi }}{T_{\mathrm{speed}}}$
      | Automatically generated on 2025-10-31 19:00:21 .
  State_w_SG_D_2_a6fad : Inport
  State_T_m_SG_D_2_ffd37 : Inport  Port=2
  Add_34d79 : Sum
  Add_405ad : Sum
  Constant_-1_ccfeb : Constant  Value=-1
  Constant_2.0_2c510 : Constant  Value=2.0
  Constant_SpeedPara_73a7d : Constant  Value=SpeedPara
  Constant_T_0_64062 : Constant  Value=T_0
  Constant_T_speed_92f50 : Constant  Value=T_speed
  Constant_f0_d5ebb : Constant  Value=f0
  Constant_pi_d0115 : Constant  Value=pi
  Constant_w_ref_ba2ef : Constant  Value=w_ref
  Divide_a38aa : Product  Inputs=*/
  Divide_c9b14 : Product  Inputs=*/
  Product_2a2b0 : Product
  Product_9a5ea : Product
  Product_da67a : Product
  Product_de508 : Product
  Subtract_0a446 : Sum  Inputs=+-
  Blockout_d_T_m_SG_D_2_41985 : Outport
  wires:
  Constant_pi_d0115/1 -> Product_2a2b0/2
  Constant_-1_ccfeb/1 -> Product_de508/1
  Constant_w_ref_ba2ef/1 -> Add_34d79/2
  State_w_SG_D_2_a6fad/1 -> Product_de508/2
  Product_de508/1 -> Add_34d79/1
  Add_405ad/1 -> Subtract_0a446/1
  Add_34d79/1 -> Product_9a5ea/2
  Constant_2.0_2c510/1 -> Product_2a2b0/1
  Constant_SpeedPara_73a7d/1 -> Product_9a5ea/1
  Product_2a2b0/1 -> Product_da67a/1
  Constant_f0_d5ebb/1 -> Product_da67a/2
  Product_9a5ea/1 -> Divide_c9b14/1
  Product_da67a/1 -> Divide_c9b14/2
  Divide_c9b14/1 -> Add_405ad/1
  Constant_T_0_64062/1 -> Add_405ad/2
  State_T_m_SG_D_2_ffd37/1 -> Subtract_0a446/2
  Subtract_0a446/1 -> Divide_a38aa/1
  Constant_T_speed_92f50/1 -> Divide_a38aa/2
  Divide_a38aa/1 -> Blockout_d_T_m_SG_D_2_41985/1

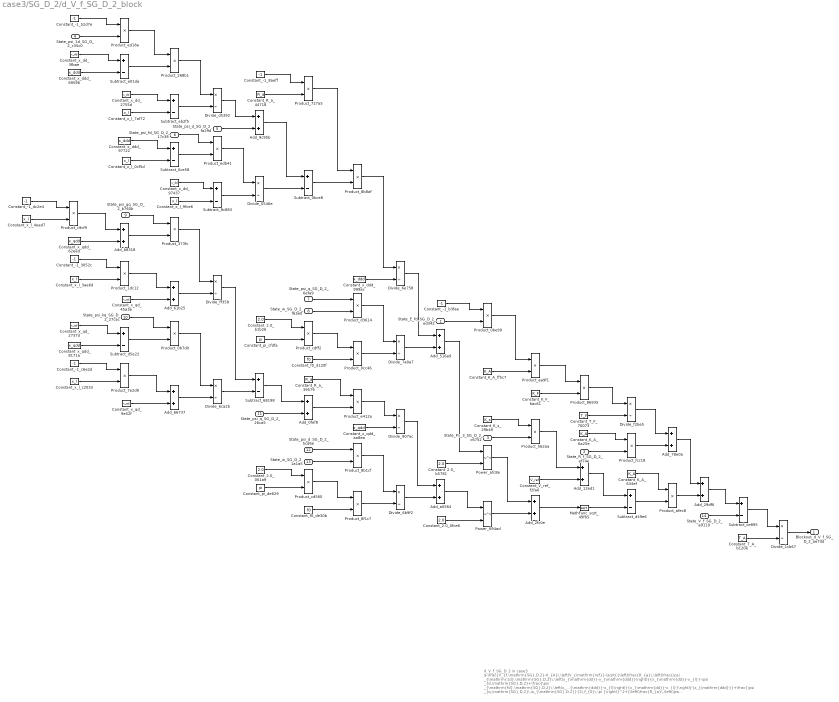
== system case3/SG_D_2/d_V_f_SG_D_2_block ==
  note: d_V_f_SG_D_2 in case3
      | $-\frac{V_{f,\mathrm{SG},D,2}-K_{A}\,\left(V_{\mathrm{ref}}-\sqrt{{\left(\frac{R_{a}\,\left(\frac{\psi _{\mathrm{1d},\mathrm{SG},D,2}\,\left(x_{\mathrm{dd}}-x_{\mathrm{ddd}}\right)}{x_{\mathrm{dd}}-x_{l}}-\psi _{d,\mathrm{SG},D,2}+\frac{\psi _{\mathrm{fd},\mathrm{SG},D,2}\,\left(x_{\mathrm{ddd}}-x_{l}\right)}{x_{\mathrm{dd}}-x_{l}}\right)}{x_{\mathrm{ddd}}}+\frac{\psi _{q,\mathrm{SG},D,2}\,w_{\mathrm{SG},D,2}}{2\,f_{0}\,\pi }\right)}^2+{\left(\frac{R_{a}\,\left(\psi _{q,\mathrm{SG},D,2}+\frac{\psi _{\mathrm{gq},\mathrm{SG},D,2}\,\left(x_{l}-x_{\mathrm{qdd}}\right)}{x_{l}-x_{\mathrm{qd}}}+\frac{\psi _{\mathrm{kq},\mathrm{SG},D,2}\,\left(x_{\mathrm{qd}}-x_{\mathrm{qdd}}\right)}{x_{l}-x_{\mathrm{qd}}}\right)}{x_{\mathrm{qdd}}}+\frac{\psi _{d,\mathrm{SG},D,2}\,w_{\mathrm{SG},D,2}}{2\,f_{0}\,\pi }\right)}^2}+K_{s}\,\mathrm{Px}_{3,\mathrm{SG},D,2}\right)-K_{A}\,R_{f,\mathrm{SG},D,2}+\frac{E_{\mathrm{fd},\mathrm{SG},D,2}\,K_{A}\,K_{F}}{T_{F}}}{T_{A}}$
      | Automatically generated on 2025-10-31 19:00:24 .
  State_E_fd_SG_D_2_ed342 : Inport
  State_R_f_SG_D_2_ef74e : Inport  Port=2
  State_Px_3_SG_D_2_c6752 : Inport  Port=3
  State_psi_1d_SG_D_2_c35c0 : Inport  Port=4
  State_psi_d_SG_D_2_fa29d : Inport  Port=5
  State_psi_fd_SG_D_2_17c38 : Inport  Port=6
  State_psi_q_SG_D_2_6efa9 : Inport  Port=7
  State_w_SG_D_2_f63e0 : Inport  Port=8
  State_psi_gq_SG_D_2_b760b : Inport  Port=9
  State_psi_kq_SG_D_2_27cac : Inport  Port=10
  State_psi_q_SG_D_2_26ca5 : Inport  Port=11
  State_psi_d_SG_D_2_5cd6e : Inport  Port=12
  State_w_SG_D_2_1a1a5 : Inport  Port=13
  State_V_f_SG_D_2_a9119 : Inport  Port=14
  Add_0fef8 : Sum
  Add_12ed1 : Sum
  Add_29df6 : Sum
  Add_2fc0e : Sum
  Add_516a9 : Sum
  Add_61b25 : Sum
  Add_66737 : Sum
  Add_78e0a : Sum
  Add_9c95b : Sum
  Add_a0564 : Sum
  Add_b8318 : Sum
  Constant_-1_3052c : Constant  Value=-1
  Constant_-1_52d7e : Constant  Value=-1
  Constant_-1_8aeff : Constant  Value=-1
  Constant_-1_b3fae : Constant  Value=-1
  Constant_-1_c6e2d : Constant  Value=-1
  Constant_-1_dc2e4 : Constant  Value=-1
  Constant_2.0_061a9 : Constant  Value=2.0
  Constant_2.0_0fce6 : Constant  Value=2.0
  Constant_2.0_b1b26 : Constant  Value=2.0
  Constant_2.0_b5781 : Constant  Value=2.0
  Constant_K_A_634ef : Constant  Value=K_A
  Constant_K_A_6a25e : Constant  Value=K_A
  Constant_K_A_ff5c7 : Constant  Value=K_A
  Constant_K_F_6ac61 : Constant  Value=K_F
  Constant_K_s_29b49 : Constant  Value=K_s
  Constant_R_a_39579 : Constant  Value=R_a
  Constant_R_a_44718 : Constant  Value=R_a
  Constant_T_A_b120e : Constant  Value=T_A
  Constant_T_F_70073 : Constant  Value=T_F
  Constant_V_ref_f2fa6 : Constant  Value=V_ref
  Constant_f0_d120f : Constant  Value=f0
  Constant_f0_de30b : Constant  Value=f0
  Constant_pi_cfdfa : Constant  Value=pi
  Constant_pi_de629 : Constant  Value=pi
  Constant_x_dd_2755d : Constant  Value=x_dd
  Constant_x_dd_3fbae : Constant  Value=x_dd
  Constant_x_dd_97437 : Constant  Value=x_dd
  Constant_x_ddd_69596 : Constant  Value=x_ddd
  Constant_x_ddd_97722 : Constant  Value=x_ddd
  Constant_x_ddd_999ac : Constant  Value=x_ddd
  Constant_x_l_0cf5d : Constant  Value=x_l
  Constant_x_l_3ae6d : Constant  Value=x_l
  Constant_x_l_4ead7 : Constant  Value=x_l
  Constant_x_l_7af72 : Constant  Value=x_l
  Constant_x_l_9fce6 : Constant  Value=x_l
  Constant_x_l_c2033 : Constant  Value=x_l
  Constant_x_qd_2737d : Constant  Value=x_qd
  Constant_x_qd_45a3e : Constant  Value=x_qd
  Constant_x_qd_9e52f : Constant  Value=x_qd
  Constant_x_qdd_62eed : Constant  Value=x_qdd
  Constant_x_qdd_8171a : Constant  Value=x_qdd
  Constant_x_qdd_aa8ea : Constant  Value=x_qdd
  Divide_0546e : Product  Inputs=*/
  Divide_1cb67 : Product  Inputs=*/
  Divide_6b9f2 : Product  Inputs=*/
  Divide_6ca2b : Product  Inputs=*/
  Divide_6e758 : Product  Inputs=*/
  Divide_7a0a7 : Product  Inputs=*/
  Divide_907ac : Product  Inputs=*/
  Divide_d5392 : Product  Inputs=*/
  Divide_f2be5 : Product  Inputs=*/
  Divide_ff358 : Product  Inputs=*/
  MathFunc_sqrt_49fb5 : Sqrt
  Power_694ad : Math  Operator=pow
  Power_afc8e : Math  Operator=pow
  Product_0b7d0 : Product
  Product_0be99 : Product
  Product_0cc46 : Product
  Product_1dc12 : Product
  Product_268b1 : Product
  Product_373fc : Product
  Product_562aa : Product
  Product_727a5 : Product
  Product_7e2d9 : Product
  Product_86935 : Product
  Product_8b1cf : Product
  Product_8b8af : Product
  Product_8f1c7 : Product
  Product_aa9f1 : Product
  Product_afec8 : Product
  Product_c9cf9 : Product
  Product_cd560 : Product
  Product_cdff2 : Product
  Product_d3614 : Product
  Product_e412a : Product
  Product_ed18a : Product
  Product_edb41 : Product
  Product_fcc18 : Product
  Subtract_0bce8 : Sum  Inputs=+-
  Subtract_0ce58 : Sum  Inputs=+-
  Subtract_68198 : Sum  Inputs=+-
  Subtract_8c883 : Sum  Inputs=+-
  Subtract_ce895 : Sum  Inputs=+-
  Subtract_d49e6 : Sum  Inputs=+-
  Subtract_d5e22 : Sum  Inputs=+-
  Subtract_e01da : Sum  Inputs=+-
  Subtract_eb2f5 : Sum  Inputs=+-
  Blockout_d_V_f_SG_D_2_ae7dd : Outport
  wires:
  Constant_-1_52d7e/1 -> Product_ed18a/1
  Constant_2.0_b1b26/1 -> Product_cdff2/1
  Constant_-1_dc2e4/1 -> Product_c9cf9/1
  Product_cdff2/1 -> Product_0cc46/1
  Product_c9cf9/1 -> Add_b8318/1
  Constant_x_l_c2033/1 -> Product_7e2d9/2
  Constant_x_l_4ead7/1 -> Product_c9cf9/2
  State_psi_1d_SG_D_2_c35c0/1 -> Product_ed18a/2
  Constant_x_l_9fce6/1 -> Subtract_8c883/2
  Constant_x_dd_3fbae/1 -> Subtract_e01da/1
  Product_e412a/1 -> Divide_907ac/1
  Constant_x_ddd_69596/1 -> Subtract_e01da/2
  Constant_x_qd_9e52f/1 -> Add_66737/2
  Add_b8318/1 -> Product_373fc/2
  Constant_x_qdd_62eed/1 -> Add_b8318/2
  Constant_-1_3052c/1 -> Product_1dc12/1
  Constant_x_dd_97437/1 -> Subtract_8c883/1
  Subtract_68198/1 -> Add_0fef8/1
  Power_afc8e/1 -> Add_2fc0e/1
  Constant_x_l_3ae6d/1 -> Product_1dc12/2
  Constant_2.0_061a9/1 -> Product_cd560/1
  Constant_x_qd_2737d/1 -> Subtract_d5e22/1
  Constant_pi_de629/1 -> Product_cd560/2
  Subtract_0bce8/1 -> Product_8b8af/2
  Constant_x_qdd_8171a/1 -> Subtract_d5e22/2
  State_psi_fd_SG_D_2_17c38/1 -> Product_edb41/1
  Constant_-1_c6e2d/1 -> Product_7e2d9/1
  Product_ed18a/1 -> Product_268b1/1
  State_w_SG_D_2_1a1a5/1 -> Product_8b1cf/2
  Subtract_e01da/1 -> Product_268b1/2
  Constant_x_dd_2755d/1 -> Subtract_eb2f5/1
  State_psi_q_SG_D_2_26ca5/1 -> Add_0fef8/2
  State_w_SG_D_2_f63e0/1 -> Product_d3614/2
  Subtract_0ce58/1 -> Product_edb41/2
  Constant_x_l_7af72/1 -> Subtract_eb2f5/2
  Add_78e0a/1 -> Add_29df6/1
  Constant_x_ddd_97722/1 -> Subtract_0ce58/1
  Constant_x_l_0cf5d/1 -> Subtract_0ce58/2
  State_psi_gq_SG_D_2_b760b/1 -> Product_373fc/1
  Product_1dc12/1 -> Add_61b25/1
  Subtract_8c883/1 -> Divide_0546e/2
  Constant_x_qd_45a3e/1 -> Add_61b25/2
  Product_d3614/1 -> Divide_7a0a7/1
  State_psi_kq_SG_D_2_27cac/1 -> Product_0b7d0/1
  Subtract_d5e22/1 -> Product_0b7d0/2
  Product_edb41/1 -> Divide_0546e/1
  State_V_f_SG_D_2_a9119/1 -> Subtract_ce895/2
  Product_7e2d9/1 -> Add_66737/1
  Product_268b1/1 -> Divide_d5392/1
  Divide_ff358/1 -> Subtract_68198/1
  Subtract_eb2f5/1 -> Divide_d5392/2
  Product_373fc/1 -> Divide_ff358/1
  Add_61b25/1 -> Divide_ff358/2
  Product_0b7d0/1 -> Divide_6ca2b/1
  Divide_0546e/1 -> Subtract_0bce8/2
  Constant_f0_d120f/1 -> Product_0cc46/2
  Add_66737/1 -> Divide_6ca2b/2
  Divide_d5392/1 -> Add_9c95b/1
  State_psi_d_SG_D_2_fa29d/1 -> Add_9c95b/2
  Divide_6ca2b/1 -> Subtract_68198/2
  Constant_-1_8aeff/1 -> Product_727a5/1
  Constant_R_a_44718/1 -> Product_727a5/2
  Constant_f0_de30b/1 -> Product_8f1c7/2
  Add_9c95b/1 -> Subtract_0bce8/1
  Product_727a5/1 -> Product_8b8af/1
  Constant_pi_cfdfa/1 -> Product_cdff2/2
  State_psi_q_SG_D_2_6efa9/1 -> Product_d3614/1
  Constant_R_a_39579/1 -> Product_e412a/1
  State_E_fd_SG_D_2_ed342/1 -> Product_0be99/2
  Add_0fef8/1 -> Product_e412a/2
  State_psi_d_SG_D_2_5cd6e/1 -> Product_8b1cf/1
  Product_cd560/1 -> Product_8f1c7/1
  Product_8b8af/1 -> Divide_6e758/1
  Constant_x_ddd_999ac/1 -> Divide_6e758/2
  Product_0cc46/1 -> Divide_7a0a7/2
  Constant_x_qdd_aa8ea/1 -> Divide_907ac/2
  Product_8b1cf/1 -> Divide_6b9f2/1
  Product_8f1c7/1 -> Divide_6b9f2/2
  Divide_6e758/1 -> Add_516a9/1
  Divide_7a0a7/1 -> Add_516a9/2
  Divide_907ac/1 -> Add_a0564/1
  Divide_6b9f2/1 -> Add_a0564/2
  Constant_-1_b3fae/1 -> Product_0be99/1
  Add_516a9/1 -> Power_afc8e/1
  Constant_2.0_b5781/1 -> Power_afc8e/2
  Add_a0564/1 -> Power_694ad/1
  Constant_2.0_0fce6/1 -> Power_694ad/2
  Product_0be99/1 -> Product_aa9f1/1
  Constant_K_A_ff5c7/1 -> Product_aa9f1/2
  Constant_K_s_29b49/1 -> Product_562aa/1
  State_Px_3_SG_D_2_c6752/1 -> Product_562aa/2
  Power_694ad/1 -> Add_2fc0e/2
  Product_aa9f1/1 -> Product_86935/1
  Constant_K_F_6ac61/1 -> Product_86935/2
  Product_562aa/1 -> Add_12ed1/1
  Constant_V_ref_f2fa6/1 -> Add_12ed1/2
  Add_2fc0e/1 -> MathFunc_sqrt_49fb5/1
  Product_86935/1 -> Divide_f2be5/1
  Constant_T_F_70073/1 -> Divide_f2be5/2
  Constant_K_A_6a25e/1 -> Product_fcc18/1
  State_R_f_SG_D_2_ef74e/1 -> Product_fcc18/2
  Add_12ed1/1 -> Subtract_d49e6/1
  MathFunc_sqrt_49fb5/1 -> Subtract_d49e6/2
  Divide_f2be5/1 -> Add_78e0a/1
  Product_fcc18/1 -> Add_78e0a/2
  Constant_K_A_634ef/1 -> Product_afec8/1
  Subtract_d49e6/1 -> Product_afec8/2
  Product_afec8/1 -> Add_29df6/2
  Add_29df6/1 -> Subtract_ce895/1
  Subtract_ce895/1 -> Divide_1cb67/1
  Constant_T_A_b120e/1 -> Divide_1cb67/2
  Divide_1cb67/1 -> Blockout_d_V_f_SG_D_2_ae7dd/1

== system case3/SG_D_2/d_psi_1d_SG_D_2_block ==
  note: d_psi_1d_SG_D_2 in case3
      | $-\frac{\psi _{\mathrm{1d},\mathrm{SG},D,2}-\psi _{\mathrm{fd},\mathrm{SG},D,2}+\frac{\left(x_{\mathrm{dd}}-x_{l}\right)\,\left(\frac{\psi _{\mathrm{1d},\mathrm{SG},D,2}\,\left(x_{\mathrm{dd}}-x_{\mathrm{ddd}}\right)}{x_{\mathrm{dd}}-x_{l}}-\psi _{d,\mathrm{SG},D,2}+\frac{\psi _{\mathrm{fd},\mathrm{SG},D,2}\,\left(x_{\mathrm{ddd}}-x_{l}\right)}{x_{\mathrm{dd}}-x_{l}}\right)}{x_{\mathrm{ddd}}}}{T_{\mathrm{ddd}}}$
      | Automatically generated on 2025-10-31 19:00:03 .
  State_psi_1d_SG_D_2_b7293 : Inport
  State_psi_fd_SG_D_2_8ed55 : Inport  Port=2
  State_psi_1d_SG_D_2_3fe79 : Inport  Port=3
  State_psi_d_SG_D_2_4a3d7 : Inport  Port=4
  State_psi_fd_SG_D_2_5dfd6 : Inport  Port=5
  Add_3a5ff : Sum
  Add_96758 : Sum
  Add_c0422 : Sum
  Constant_-1_68c49 : Constant  Value=-1
  Constant_-1_aace1 : Constant  Value=-1
  Constant_T_ddd_016eb : Constant  Value=T_ddd
  Constant_x_dd_00ba7 : Constant  Value=x_dd
  Constant_x_dd_9633e : Constant  Value=x_dd
  Constant_x_dd_b0312 : Constant  Value=x_dd
  Constant_x_dd_ec01d : Constant  Value=x_dd
  Constant_x_ddd_3bfa1 : Constant  Value=x_ddd
  Constant_x_ddd_598b4 : Constant  Value=x_ddd
  Constant_x_ddd_755b0 : Constant  Value=x_ddd
  Constant_x_l_7d54c : Constant  Value=x_l
  Constant_x_l_8ae4c : Constant  Value=x_l
  Constant_x_l_d27e4 : Constant  Value=x_l
  Constant_x_l_fa963 : Constant  Value=x_l
  Divide_21a0d : Product  Inputs=*/
  Divide_607c7 : Product  Inputs=*/
  Divide_80e86 : Product  Inputs=*/
  Divide_dcc95 : Product  Inputs=*/
  Product_4fe40 : Product
  Product_8ce48 : Product
  Product_9a83d : Product
  Product_ba8c5 : Product
  Product_f8d0b : Product
  Subtract_04dfb : Sum  Inputs=+-
  Subtract_29beb : Sum  Inputs=+-
  Subtract_443fe : Sum  Inputs=+-
  Subtract_7413b : Sum  Inputs=+-
  Subtract_88483 : Sum  Inputs=+-
  Subtract_934a3 : Sum  Inputs=+-
  Blockout_d_psi_1d_SG_D_2_dad19 : Outport
  wires:
  Subtract_934a3/1 -> Product_8ce48/2
  Constant_x_l_fa963/1 -> Subtract_04dfb/2
  Divide_dcc95/1 -> Add_3a5ff/2
  Subtract_88483/1 -> Product_4fe40/2
  Constant_-1_aace1/1 -> Product_ba8c5/1
  Constant_x_dd_b0312/1 -> Subtract_7413b/1
  Divide_607c7/1 -> Blockout_d_psi_1d_SG_D_2_dad19/1
  State_psi_fd_SG_D_2_8ed55/1 -> Add_c0422/2
  State_psi_1d_SG_D_2_3fe79/1 -> Product_ba8c5/2
  Divide_21a0d/1 -> Subtract_88483/2
  Constant_x_ddd_3bfa1/1 -> Subtract_7413b/2
  State_psi_1d_SG_D_2_b7293/1 -> Product_f8d0b/2
  Product_ba8c5/1 -> Product_9a83d/1
  Subtract_7413b/1 -> Product_9a83d/2
  Constant_x_dd_00ba7/1 -> Subtract_04dfb/1
  Constant_x_ddd_598b4/1 -> Subtract_934a3/1
  Constant_x_l_7d54c/1 -> Subtract_934a3/2
  Product_9a83d/1 -> Divide_80e86/1
  Subtract_04dfb/1 -> Divide_80e86/2
  State_psi_fd_SG_D_2_5dfd6/1 -> Product_8ce48/1
  Constant_x_dd_9633e/1 -> Subtract_29beb/1
  Constant_x_l_d27e4/1 -> Subtract_443fe/2
  Constant_x_l_8ae4c/1 -> Subtract_29beb/2
  Constant_x_ddd_755b0/1 -> Divide_dcc95/2
  Divide_80e86/1 -> Add_96758/1
  State_psi_d_SG_D_2_4a3d7/1 -> Add_96758/2
  Product_8ce48/1 -> Divide_21a0d/1
  Subtract_29beb/1 -> Divide_21a0d/2
  Constant_x_dd_ec01d/1 -> Subtract_443fe/1
  Add_96758/1 -> Subtract_88483/1
  Constant_-1_68c49/1 -> Product_f8d0b/1
  Subtract_443fe/1 -> Product_4fe40/1
  Product_f8d0b/1 -> Add_c0422/1
  Product_4fe40/1 -> Divide_dcc95/1
  Add_c0422/1 -> Add_3a5ff/1
  Add_3a5ff/1 -> Divide_607c7/1
  Constant_T_ddd_016eb/1 -> Divide_607c7/2
